simulink model "estados"  (Simulink 8.1)
settings: Solver=ode45  StartTime=0.0  StopTime=40  RelTol=1e-3
values from neighbouring files (symbols this model uses):
  A = [0, 1, 0; 0, 0, 1; 0, -1/(tau2*tau3), -(tau2+tau3)/(tau2*tau3)]    [script.m]
  B = [0; 0; k1*k2*k3*k4/(tau2*tau3)]    [script.m]
  C = [1, 0, 0]    [script.m]
  K = place(A,B,vpc)    [script.m]
  L = transpose(acker(A',C',vpo))    [script.m]
  Sample_time = 0.001    [script.m]
libraries: cstblocks x1, simulink x1
settings Model: Creator=PhM  LastModifiedBy=dello
settings DataIOCC: LimitDataPoints=off  SignalLoggingSaveFormat=Dataset  StateSaveName=x, xest  SignalLoggingName=stateslog
settings OptimizationCC: InitFltsAndDblsToZero=on
settings DebuggingCC: SaveWithParameterizedLinksMsg=none  SignalResolutionControl=TryResolveAllWithWarning  MultiTaskDSMMsg=warning  MultiTaskCondExecSysMsg=none  StrictBusMsg=None
settings RTWCC: IncludeERTFirstTime=on
settings GRTTargetCC: TargetFcnLib=ansi_tfl_tmw.mat

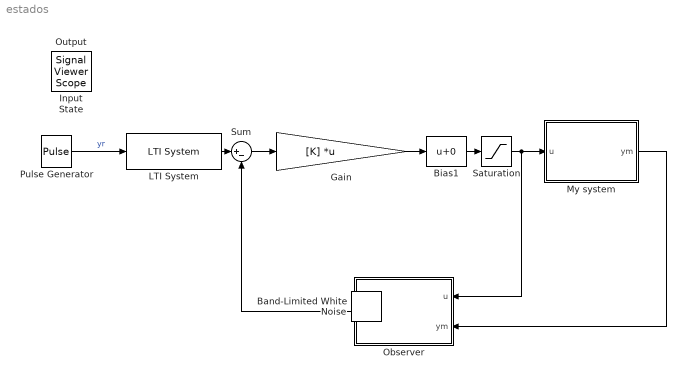
== system estados ==
  Bias1 : Bias
  Gain : Gain  Gain=[K]  Multiplication=Matrix(K*u) (u vector)
  LTI System : cstblocks/LTI System  sys=M  IC=[]
  My system : Subsystem
  Observer : Subsystem
  Pulse Generator : DiscretePulseGenerator  PulseType=Time based  Period=4  PulseWidth=50
  Saturation : Saturate  UpperLimit=10  LowerLimit=-10
  Sum : Sum  Inputs=|+-
  Band-Limited White Noise : simulink/Sources/Band-Limited White Noise  IOType=siggen  Cov=Noise_step  Ts=Sample_time  seed=[23341]
  Input : SignalViewerScope  IOType=viewer  RefreshTime=0.035000
      settings: ShowLegends=on  TimeRange=40  YMin=-0.4  YMax=0.45  SaveName=ScopeData2
  Output : SignalViewerScope  IOType=viewer  NumInputPorts=2  RefreshTime=0.035000
      settings: ShowLegends=on  TimeRange=40  YMin=-2~-2  YMax=2.25~2.25
  State : SignalViewerScope  IOType=viewer  RefreshTime=0.035000
      settings: ShowLegends=on  TimeRange=40  YMin=-0.4  YMax=0.45
  wires:
  My system/1(ym) -> Observer/2(ym)
  Gain/1 -> Bias1/1
  Sum/1 -> Gain/1
  Bias1/1 -> Saturation/1
  Pulse Generator/1 -> LTI System/1  "yr"
  Observer/1(xest) -> Sum/2
  LTI System/1 -> Sum/1
  Saturation/1 -> My system/1(u), Observer/1(u)

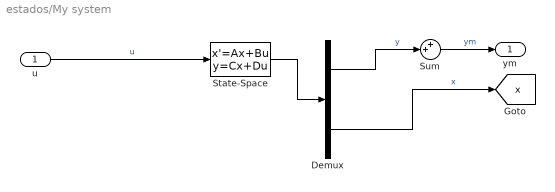
== system estados/My system ==
  u : Inport
  Demux : Demux  Outputs=[1 3]
  State-Space : StateSpace  A=A  B=B  C=[C; eye(3)]  D=zeros(4,1)  X0=zeros(3,1)
  Sum : Sum  Inputs=++|
  ym : Outport
  tag scope: x=global
  wires:
  State-Space/1 -> Demux/1
  Demux/1 -> Sum/2  "y"
  Demux/2 -> [x]  "x"
  u/1 -> State-Space/1  "u"
  Sum/1 -> ym/1  "ym"

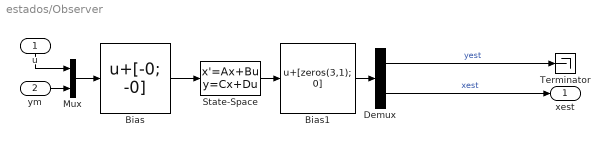
== system estados/Observer ==
  u : Inport
  ym : Inport  Port=2
  Bias : Bias  Bias=[-0; -0]
  Bias1 : Bias  Bias=[zeros(3,1); 0]
  Demux : Demux  Outputs=[1 3]
  Mux : Mux  Inputs=2
  State-Space : StateSpace  A=A-L*C  B=[B L]  C=[C; eye(3)]  D=zeros(4,2)  X0=[1; 0; 0]
  Terminator : Terminator
  xest : Outport
  wires:
  Mux/1 -> Bias/1
  State-Space/1 -> Bias1/1
  u/1 -> Mux/1
  ym/1 -> Mux/2
  Demux/1 -> Terminator/1  "yest"
  Demux/2 -> xest/1  "xest"
  Bias/1 -> State-Space/1
  Bias1/1 -> Demux/1
